simulink model "Simulink_VDP_Koopman"  (R2022a)
settings: Solver=FixedStepAuto  StartTime=0.0  StopTime=Tf  FixedStep=Ts  RelTol=1e-3
undefined symbols (not defined in the file or in its folder): A, B, X0
libraries: mpclib x1
settings Model: Creator=sergiovaneg  LastModifiedBy=sergiovaneg

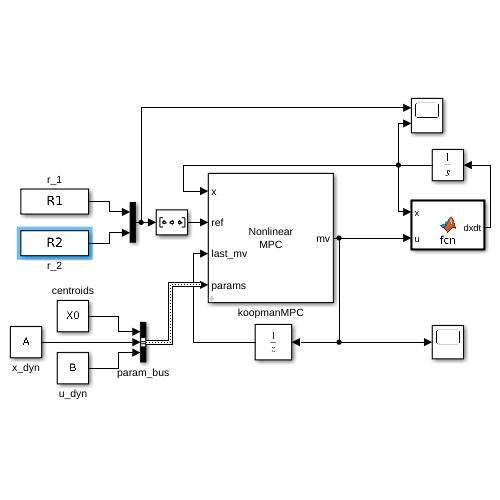
[thumbnail: Simulink's stored preview of the top-level diagram]
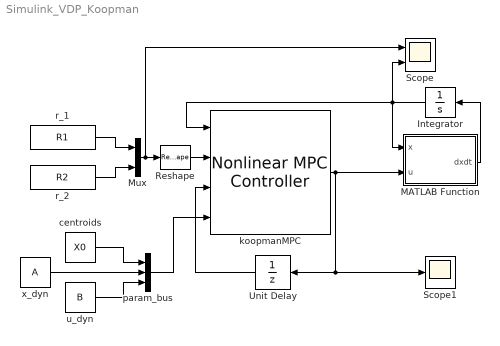
== system Simulink_VDP_Koopman ==
  Integrator : Integrator
  MATLAB Function : MATLAB Function  TreatAsAtomicUnit=on
  Mux : Mux  Inputs=2
  Reshape : Reshape  OutputDimensionality=Row vector (2-D)
  Scope : Scope  NumInputPorts=2
  Scope1 : Scope
  Unit Delay : UnitDelay  SampleTime=-1  HasFrameUpgradeWarning=on
  centroids : Constant  Value=X0
  koopmanMPC : mpclib/Nonlinear MPC Controller  nlmpcobj=nlobj  UseObjectTs=on  UseMEX=off  md_enabled=off  mvtarget_enabled=off  param_enabled=on  cost_enabled=off  mvseq_enabled=off  stateseq_enabled=off  ovseq_enabled=off  slack_enabled=off  status_enabled=off  ov_min=off  ov_max=off  mv_min=off  mv_max=off  mvrate_min=off  mvrate_max=off  state_min=off  state_max=off  ov_weight=off  mv_weight=off  mvrate_weight=off  ecr_weight=off  nlp_initialize=off
  param_bus : BusCreator  Inputs=3  OutDataTypeStr=Bus: param_bus  NonVirtualBus=on
      settings: InheritFromInputs=off
  r_1 : FromWorkspace  VariableName=R1
  r_2 : FromWorkspace  VariableName=R2
  u_dyn : Constant  Value=B
  x_dyn : Constant  Value=A
  wires:
  koopmanMPC/1 -> Unit Delay/1, Scope1/1, MATLAB Function/2(u)
  Unit Delay/1 -> koopmanMPC/3
  MATLAB Function/1(dxdt) -> Integrator/1
  Integrator/1 -> Scope/2, MATLAB Function/1(x), koopmanMPC/1
  r_1/1 -> Mux/1
  r_2/1 -> Mux/2
  Reshape/1 -> koopmanMPC/2
  Mux/1 -> Scope/1, Reshape/1
  centroids/1 -> param_bus/1
  x_dyn/1 -> param_bus/2
  u_dyn/1 -> param_bus/3
  param_bus/1 -> koopmanMPC/4

== matlab function Simulink_VDP_Koopman/MATLAB Function ==
  data: x input; u input; dxdt output
function dxdt = fcn(x,u)
    dxdt=zeros(2,1);
    dxdt(1) = 2*x(2);
    dxdt(2) = -0.8*x(1)+2*x(2)-10*(x(1)^2)*x(2) + u;
end
